simulink model "modelab1"  (R2018b)
settings: Solver=ode4  StartTime=0.0  StopTime=10.0  FixedStep=1e-2  RelTol=1e-3
values from neighbouring files (symbols this model uses):
  initval = 3    [skrpyt1.m]
  K = 1/(R*C)    (= 1)    [skrpyt1.m]
  steptime = 5    [skrpyt1.m]
  WPC = 5    [skrpyt1.m]
settings Model: Creator=student  LastModifiedBy=student

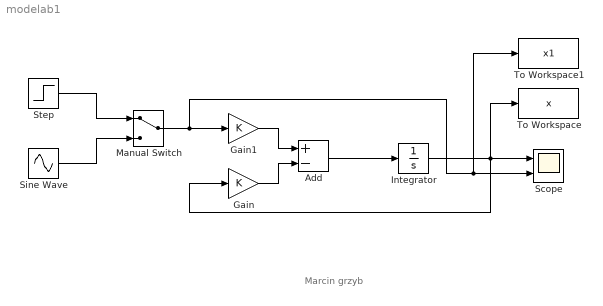
== system modelab1 ==
  note: Marcin grzyb
  Add : Sum  Inputs=+-
  Gain : Gain  Gain=K
  Gain1 : Gain  Gain=K
  Integrator : Integrator  InitialCondition=WPC
  Manual Switch : ManualSwitch
  Scope : Scope  NumInputPorts=2
  Sine Wave : Sin  Frequency=10  SampleTime=0
  Step : Step  Time=steptime  Before=initval  After=0  SampleTime=0
  To Workspace : ToWorkspace  VariableName=x  SampleTime=-1
  To Workspace1 : ToWorkspace  VariableName=x1  SampleTime=-1
  wires:
  Step/1 -> Manual Switch/1
  Sine Wave/1 -> Manual Switch/2
  Manual Switch/1 -> To Workspace1/1, Scope/2, Gain1/1
  Gain1/1 -> Add/1
  Gain/1 -> Add/2
  Add/1 -> Integrator/1
  Integrator/1 -> To Workspace/1, Gain/1, Scope/1
